simulink model "es5_sim_MODSIM"  (R2025b)
settings: Solver=VariableStepAuto  StartTime=0.0  StopTime=100  RelTol=1e-3
values from neighbouring files (symbols this model uses):
  ueq = 0.5    [es5_MODSIM.m]    (also in es5_mio.m)
  x0 = [10,10]'    [es5_MODSIM.m]    (also in es5_mio.m)
  ys = 80    [es5_MODSIM.m]
settings Model: Creator=robert  LastModifiedBy=robert

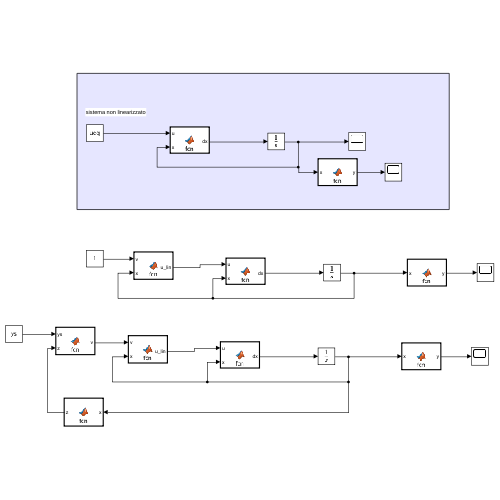
[thumbnail: Simulink's stored preview of the top-level diagram]
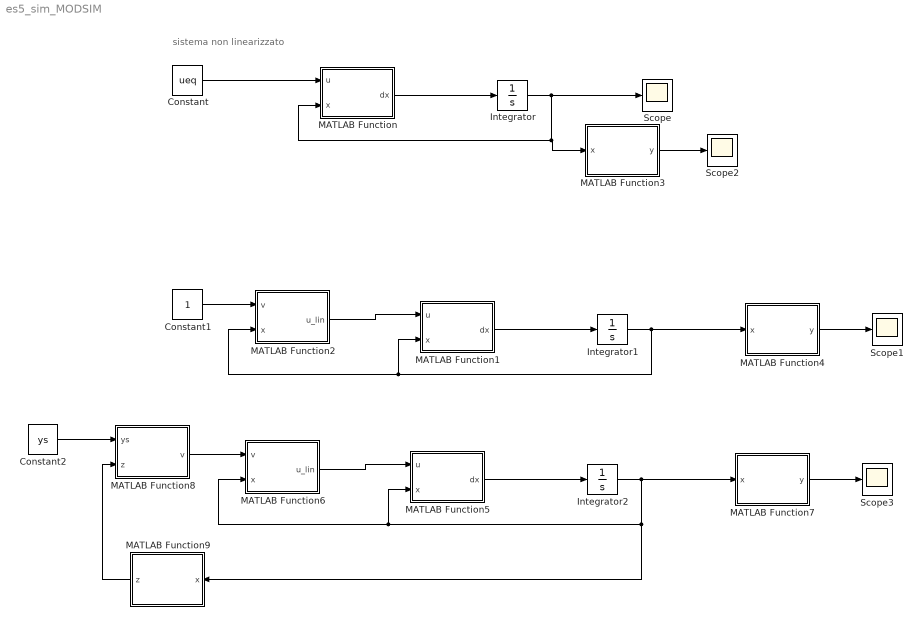
== system es5_sim_MODSIM ==
  note: sistema non linearizzato
  Constant : Constant  Value=ueq
  Constant1 : Constant
  Constant2 : Constant  Value=ys
  Integrator : Integrator  InitialCondition=x0
  Integrator1 : Integrator  InitialCondition=x0
  Integrator2 : Integrator  InitialCondition=x0
  MATLAB Function : MATLAB Function  TreatAsAtomicUnit=on
  MATLAB Function1 : MATLAB Function  TreatAsAtomicUnit=on
  MATLAB Function2 : MATLAB Function  TreatAsAtomicUnit=on
  MATLAB Function3 : MATLAB Function  TreatAsAtomicUnit=on
  MATLAB Function4 : MATLAB Function  TreatAsAtomicUnit=on
  MATLAB Function5 : MATLAB Function  TreatAsAtomicUnit=on
  MATLAB Function6 : MATLAB Function  TreatAsAtomicUnit=on
  MATLAB Function7 : MATLAB Function  TreatAsAtomicUnit=on
  MATLAB Function8 : MATLAB Function  TreatAsAtomicUnit=on
  MATLAB Function9 : MATLAB Function  TreatAsAtomicUnit=on
  Scope{,1..3} (4 alike) : Scope
      Scope settings: ActiveDisplayYMinimum=0.72328479272570512  ActiveDisplayYMaximum=87.4955730690346
      Scope1 settings: ActiveDisplayYMinimum=-1  ActiveDisplayYMaximum=1
      Scope2 settings: ActiveDisplayYMinimum=0.72328479272570512  ActiveDisplayYMaximum=87.4955730690346  DataLoggingVariableName=ScopeData2
      Scope3 settings: ActiveDisplayYMinimum=1.2506184849193485  ActiveDisplayYMaximum=88.744433635725883  DataLoggingVariableName=ScopeData3
  wires:
  MATLAB Function/1(dx) -> Integrator/1
  Integrator/1 -> Scope/1, MATLAB Function3/1(x), MATLAB Function/2(x)
  Constant/1 -> MATLAB Function/1(u)
  MATLAB Function1/1(dx) -> Integrator1/1
  Integrator1/1 -> MATLAB Function4/1(x), MATLAB Function1/2(x), MATLAB Function2/2(x)
  MATLAB Function2/1(u_lin) -> MATLAB Function1/1(u)
  MATLAB Function3/1(y) -> Scope2/1
  Constant1/1 -> MATLAB Function2/1(v)
  MATLAB Function4/1(y) -> Scope1/1
  MATLAB Function5/1(dx) -> Integrator2/1
  Integrator2/1 -> MATLAB Function7/1(x), MATLAB Function9/1(x), MATLAB Function5/2(x), MATLAB Function6/2(x)
  MATLAB Function7/1(y) -> Scope3/1
  MATLAB Function8/1(v) -> MATLAB Function6/1(v)
  MATLAB Function6/1(u_lin) -> MATLAB Function5/1(u)
  Constant2/1 -> MATLAB Function8/1(ys)
  MATLAB Function9/1(z) -> MATLAB Function8/2(z)

== matlab function es5_sim_MODSIM/MATLAB Function ==
  data: u input; dx output; x input
function dx = fcn(u, x)

alfa1= 0.02;
alfa2 = 0.001;
K = 100;
b = 0.1;
x1 = x(1);
x2 = x(2);

dx = [x1 * (1 - x1/K) - alfa1 * x1 * x2; -b * x2 + alfa2 * x1 * x2 + u];

== matlab function es5_sim_MODSIM/MATLAB Function2 ==
  data: v input; u_lin output; x input
function u_lin = fcn(v,x)

x1 = x(1);
x2 = x(2);

u_lin = (10*x1^3 + 29*x1^2*x2 - 1500*x1^2 + 20*x1*x2^2 - 1900*x1*x2 + 50000*x1 - 50000*v)/(1000*x1);

== matlab function es5_sim_MODSIM/MATLAB Function3 ==
  data: y output; x input
function y = fcn(x)

y = x(1);

== matlab function es5_sim_MODSIM/MATLAB Function4 ==
  data: y output; x input
function y = fcn(x)

y = x(1);

== matlab function es5_sim_MODSIM/MATLAB Function5 ==
  data: u input; dx output; x input
function dx = fcn(u, x)

alfa1= 0.02;
alfa2 = 0.001;
K = 100;
b = 0.1;
x1 = x(1);
x2 = x(2);

dx = [x1 * (1 - x1/K) - alfa1 * x1 * x2; -b * x2 + alfa2 * x1 * x2 + u];

== matlab function es5_sim_MODSIM/MATLAB Function6 ==
  data: v input; u_lin output; x input
function u_lin = fcn(v,x)

x1 = x(1);
x2 = x(2);

u_lin = (10*x1^3 + 29*x1^2*x2 - 1500*x1^2 + 20*x1*x2^2 - 1900*x1*x2 + 50000*x1 - 50000*v)/(1000*x1);

== matlab function es5_sim_MODSIM/MATLAB Function7 ==
  data: y output; x input
function y = fcn(x)

y = x(1);

== matlab function es5_sim_MODSIM/MATLAB Function8 ==
  data: ys input; v output; z input
function v = fcn(ys,z)

z1 = z(1);
z2 = z(2);
K = [1.0000 10.1000]

v = -K(1)*z1 - K(2)*z2 + K(1)*ys;

== matlab function es5_sim_MODSIM/MATLAB Function9 ==
  data: x input; z output
function z = fcn(x)

x1 = x(1);
x2 = x(2);

z =[x1; - x1*(x1/100 - 1) - (x1*x2)/50];

== matlab function es5_sim_MODSIM/MATLAB Function1 ==
  data: u input; dx output; x input
function dx = fcn(u, x)

alfa1= 0.02;
alfa2 = 0.001;
K = 100;
b = 0.1;
x1 = x(1);
x2 = x(2);

dx = [x1 * (1 - x1/K) - alfa1 * x1 * x2; -b * x2 + alfa2 * x1 * x2 + u];
